simulink model "simu"  (R2021a)
settings: Solver=VariableStepAuto  StartTime=0.0  StopTime=48387  RelTol=1e-3
libraries: simulink x1
settings Model: Creator=jricl  LastModifiedBy=jricl

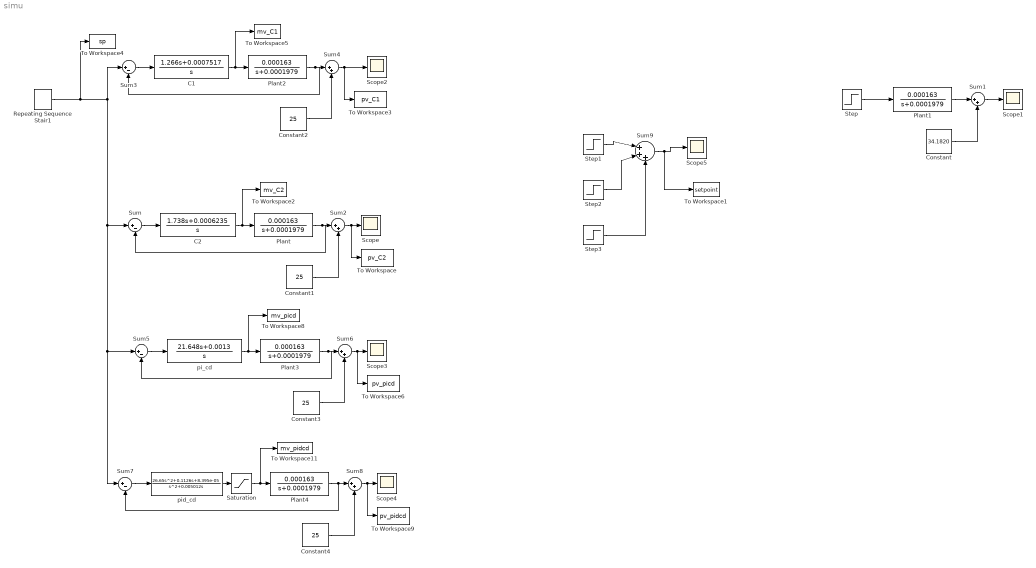
== system simu ==
  C1 : TransferFcn  Numerator="[1.266  0.0007517]"  Denominator=[1 0]
  C2 : TransferFcn  Numerator="[1.738  0.0006235]"  Denominator=[1 0]
  Constant : Constant  Value=34.1820
  Constant{1..4} (4 alike) : Constant  Value=25
  Plant{,1..4} (5 alike) : TransferFcn  Numerator=[0.000163]  Denominator=[1 0.0001979]
  Repeating Sequence Stair1 : simulink/Sources/Repeating Sequence Stair  OutValues=[5 10 15 20]  tsamp=25000  OutMin=[]  OutMax=[]  OutDataTypeStr=double  OutputDataTypeScalingMode=double  OutDataType=fixdt(0,8)  ConRadixGroup=Best Precision: Vector-wise  OutScaling=2^-12
  Saturation : Saturate  UpperLimit=100  LowerLimit=0
  Scope{,1..5} (6 alike) : Scope
  Step : Step  Time=0  After=2  SampleTime=1
  Step1 : Step  Time=25000  Before=30  After=35
  Step2 : Step  Time=25000+25000  After=5
  Step3 : Step  Time=25000+25000+25000  After=5
  Sum{,3,5,7} (4 alike) : Sum  Inputs=|+-
  Sum{1..2,4,6,8} (5 alike) : Sum  Inputs=|++
  Sum9 : Sum  Inputs=|+++
  To Workspace : ToWorkspace  VariableName=pv_C2  SaveFormat=Timeseries  SampleTime=-1
  To Workspace1 : ToWorkspace  VariableName=setpoint  SaveFormat=Timeseries  SampleTime=-1
  To Workspace11 : ToWorkspace  VariableName=mv_pidcd  SaveFormat=Timeseries  SampleTime=-1
  To Workspace2 : ToWorkspace  VariableName=mv_C2  SaveFormat=Timeseries  SampleTime=-1
  To Workspace3 : ToWorkspace  VariableName=pv_C1  SaveFormat=Timeseries  SampleTime=-1
  To Workspace4 : ToWorkspace  VariableName=sp  SaveFormat=Timeseries  SampleTime=-1
  To Workspace5 : ToWorkspace  VariableName=mv_C1  SaveFormat=Timeseries  SampleTime=-1
  To Workspace6 : ToWorkspace  VariableName=pv_picd  SaveFormat=Timeseries  SampleTime=-1
  To Workspace8 : ToWorkspace  VariableName=mv_picd  SaveFormat=Timeseries  SampleTime=-1
  To Workspace9 : ToWorkspace  VariableName=pv_pidcd  SaveFormat=Timeseries  SampleTime=-1
  pi_cd : TransferFcn  Numerator="[21.648  0.0013]"  Denominator=[1 0]
  pid_cd : TransferFcn  Numerator=[26.65 0.1126 8.395e-05]  Denominator=[1 0.005012 0]
  wires:
  Plant/1 -> Sum/2, Sum2/1
  Sum/1 -> C2/1
  Step/1 -> Plant1/1
  Plant1/1 -> Sum1/1
  Sum1/1 -> Scope1/1
  Constant/1 -> Sum1/2
  C2/1 -> To Workspace2/1, Plant/1
  Sum2/1 -> To Workspace/1, Scope/1
  Constant1/1 -> Sum2/2
  Constant2/1 -> Sum4/2
  Sum4/1 -> Scope2/1, To Workspace3/1
  C1/1 -> Plant2/1, To Workspace5/1
  Sum3/1 -> C1/1
  Plant2/1 -> Sum4/1, Sum3/2
  Plant3/1 -> Sum5/2, Sum6/1
  Sum5/1 -> pi_cd/1
  pi_cd/1 -> To Workspace8/1, Plant3/1
  Sum6/1 -> To Workspace6/1, Scope3/1
  Constant3/1 -> Sum6/2
  Constant4/1 -> Sum8/2
  Sum8/1 -> Scope4/1, To Workspace9/1
  Sum7/1 -> pid_cd/1
  Plant4/1 -> Sum8/1, Sum7/2
  Repeating Sequence Stair1/1 -> To Workspace4/1, Sum3/1, Sum7/1, Sum5/1, Sum/1
  Step1/1 -> Sum9/1
  Step2/1 -> Sum9/2
  Sum9/1 -> To Workspace1/1, Scope5/1
  Step3/1 -> Sum9/3
  pid_cd/1 -> Saturation/1
  Saturation/1 -> To Workspace11/1, Plant4/1
